simulink library "basic_create_THB"  (R2016b)
settings: Solver=ode45  StartTime=0.0  StopTime=10.0  RelTol=1e-3  EnableMultiTasking=on
undefined symbols (not defined in the file): Water
libraries: carnot x3
settings Model: Creator=lena.frank  LastModifiedBy=awohlfei
settings DataIOCC: LimitDataPoints=on  SaveFormat=Array  SignalLoggingSaveFormat=ModelDataLogs
settings OptimizationCC: ExpressionDepthLimit=2147483647  LifeSpan=inf
settings DebuggingCC: UnderspecifiedInitializationDetection=Classic  MergeDetectMultiDrivingBlocksExec=none  SolverPrmCheckMsg=warning  FcnCallInpInsideContextMsg=warning  StateNameClashWarn=warning  SFUnexpectedBacktrackingDiag=warning  SFNoUnconditionalDefaultTransitionDiag=warning  SFExecutionAtInitializationDiag=none
settings HardwareCC: ProdBitPerPointer=32  ProdBitPerSizeT=32  ProdBitPerPtrDiffT=32  ProdLargestAtomicFloat=None  ProdIntDivRoundTo=Undefined  ProdEndianess=Unspecified  ProdWordSize=32  ProdHWDeviceType=32-bit Generic
settings ModelReferenceCC: PropagateSignalLabelsOutOfModel=off
settings GRTTargetCC: TargetLangStandard=C89/C90 (ANSI)  GeneratePreprocessorConditionals=Disable all  CombineOutputUpdateFcns=off  GRTInterface=on
settings ConfigComp: CovMetricSettings=dw  CovHtmlReporting=on  CovSaveCumulativeToWorkspaceVar=on  CovSaveSingleToWorkspaceVar=on  CovExternalEMLEnable=off

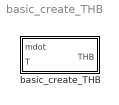
== system basic_create_THB ==
  basic_create_THB : Subsystem  InitFcn=load('THB.mat');  mask(basic create THB){p=1e5, fluid=Water, mix=0, mix2=0, mix3=0, dia=0.02, hgt=0, mID=No Pressure Drop}
      mask prompts: p "pressure [Pa]"; mix "fluid mixture [0..1]"; mix2 "fluid mixture 2 [0..1]"; mix3 "fluid mixture 3 [0..1]"; dia "diameter [m]"; hgt "Static height in m"; mID "ID for pressure drop calculation"
      mask help:
      | Create a THB with the variable input T and mdot. The other value can be set as constants in the mask.
      | Pressure drop calculation mode (defined by ID):
      |     1 ..  9999 no pressure drop (dp)
      | 10001 .. 19999 dp caused by flowrate
      | 20001 .. inf   dp by flowrate and static height
      mask init:
      | mix = min(1, max(0, mix));
      | dia = max(dia, 0.001);
      mask Help: web(fullfile(path_carnot('help'),'basic_create_THB.html'),'-helpbrowser')
      mask TypeOptions p: basic_THB/p
      mask TypeOptions fluid: basic_THB/fluid
      mask TypeOptions mix: basic_THB/mix
      mask TypeOptions mix2: basic_THB/mix2
      mask TypeOptions mix3: basic_THB/mix3
      mask TypeOptions dia: basic_THB/dia
      mask TypeOptions hgt: basic_THB/hgt
      mask TypeOptions mID: basic_THB/ID

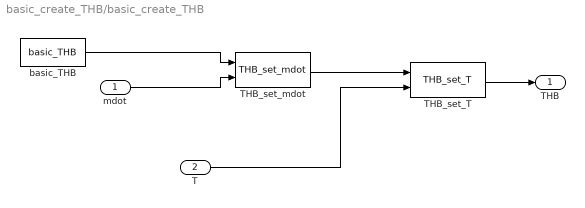
== system basic_create_THB/basic_create_THB ==
  mdot : Inport
  T : Inport  Port=2
  THB_set_T : carnot/Source/Simple/THB_set_T
  THB_set_mdot : carnot/Source/Simple/THB_set_mdot
  basic_THB : carnot/Basic/Hydraulics/basic_THB  t=10  mdot=0  p=p  ID=No Pressure Drop  fluid=Water  mix=mix  mix2=mix2  mix3=mix3  dia=dia  hgt=hgt
  THB : Outport
  wires:
  basic_THB/1 -> THB_set_mdot/1
  mdot/1 -> THB_set_mdot/2
  THB_set_mdot/1 -> THB_set_T/1
  THB_set_T/1 -> THB/1
  T/1 -> THB_set_T/2
